simulink model "qss_saab93_optigear"  (Simulink 8.8)
settings: Solver=VariableStepDiscrete  StartTime=0.0  StopTime=1220  RelTol=1e-3  EnableMultiTasking=on
undefined symbols (not defined in the file or in its folder): g, h, rho
libraries: qss_tb_library x3
settings Model: Creator=grauers  LastModifiedBy=grauers
settings OptimizationCC: InitFltsAndDblsToZero=on
settings DebuggingCC: SaveWithParameterizedLinksMsg=none  SignalResolutionControl=TryResolveAllWithWarning  SolverPrmCheckMsg=warning  MultiTaskDSMMsg=warning  MultiTaskCondExecSysMsg=none  StateNameClashWarn=none  StrictBusMsg=None
settings GRTTargetCC: TargetFcnLib=ansi_tfl_tmw.mat  GeneratePreprocessorConditionals=Use local settings

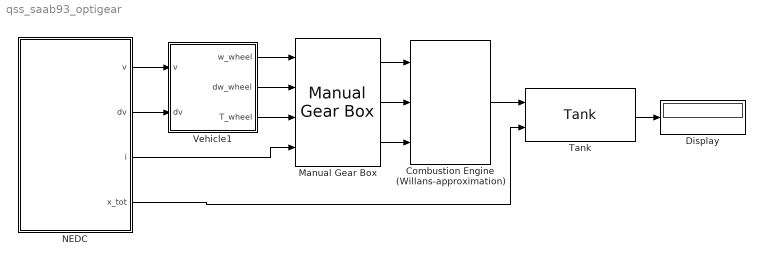
== system qss_saab93_optigear ==
  Combustion Engine (Willans-approximation) : qss_tb_library/Energy Converter/Combustion Engine (Willans-approximation)  Tag=combustion engine  engine_type=Otto  V_d=1.985  theta_CE=0.05  S=78  B=90  w_CE_idle=105  P_CE_idle=2600  P_aux=300  e=0.46  PI=1.44  p_me0g=1  ENABLE_FUEL_CUTOFF=on  T_CE_cutoff=5  P_CE_cutoff=0
  Display : Display
  Manual Gear Box : qss_tb_library/Gear System/Manual Gear Box  Tag=transmission  i_1=first_gear  i_2=second_gear  i_3=third_gear  i_4=fourth_gear  i_5=fifth_gear  i_diff=diff_gear  e_GT=0.98  P_GT0=300  w_wheel_min=1
  NEDC : Subsystem  Tag=cycle  mask(Driving Cycle){cyclename1=NEDC, stepsize=1, autostop=on}
      mask prompts: cyclename1 "Choose a cycle"; stepsize "Step size [s]"; autostop "Enable automatic simulation stop"
      mask help:
      | This block loads the cycle data such as time, speed, acceleration and gear number,  from the specified data file and makes it available on the output of the cycle block.
      |
      | Output:
      | ======
      | 	v	Speed [m/s]
      | 	dv	Acceleration [m/s^2]
      | 	i	Gear number [-]
      | 	x_tot	Total distance [m]
      |
      | Tip:
      | ===
      | Probably you don't need the gear number "i". If so you can terminate
      | it with a "Terminator" out of the "Simulink Library/Connections."
      |
      | Driving cycle:
      | ===
      | Select a driving cycle from the list below or specify your own (place your .mat file in the
      | directory Data/DrivingCycles/UserDefined)
      |
      | ECE_MAN
      | ECE_R15s
      | ECE_R15
      | EUDC
      | EUDC_MAN
      | City
      | City_MAN
      | NEDC
      | NEDC_MANl
      | GOT1
      | GOT2
      | GOT3
      | 10_15_MODE
      | 10_MODE
      | 10_MODE_3
      | 11_MODE
      | 11_MODE_4
      | 15_MODE
      | City_I
      | City_II
      | FTP_75
      | FTP_Highway
      |
      |
      | Step size:
      | ========
      | Default value is 1. Don't change it, unless you are familiar with the programs of the QSS TB.
      |
      | Enable automatic simulation stop:
      | ===========================
      | Stops the simulation automatically at the end of the cycle.
      | Be careful: If you have a component in your model that has to run after the cycle has finished, e.g. a battery to charge, remove the mark!
      mask init:
      | init_driving_cycle1;
      mask Display: plot(T_zplot, V_zplot);
  Tank : qss_tb_library/Energy Source/Tank  Tag=tank  fuel=Gasoline  flag_cold_start=on
  Vehicle1 : Subsystem  Tag=vehicle  mask(Vehicle){m_f=1295+80+100, mt2m_f=5, A_f=2, d_wheel=0.62, cw=0.3, mu=0.013}
      mask prompts: m_f "Total mass of the vehicle [kg]"; mt2m_f "Rotating mass [%]"; A_f "Vehicle cross section [m^2]"; d_wheel "Wheel diameter [m]"; cw "Drag coefficient [-]"; mu "Rolling friction coefficient [-]"
      mask help:
      | This block computes the power required from the vehicle.
      |
      | Input:
      | =====
      | 	v		Speed [m/s]
      | 	dv		Acceleration [m/s^2]
      |
      | Output:
      | ======
      | 	w_wheel	Speed of the wheel [rad/s]
      | 	dw_wheel	Acceleration of the wheel [rad/s^2]
      | 	T_wheel	Torque on the wheel [Nm]
      mask init:
      | init_vehicle;
  wires:
  NEDC/1(v) -> Vehicle1/1(v)
  Vehicle1/1(w_wheel) -> Manual Gear Box/1
  Vehicle1/2(dw_wheel) -> Manual Gear Box/2
  Vehicle1/3(T_wheel) -> Manual Gear Box/3
  NEDC/2(dv) -> Vehicle1/2(dv)
  Manual Gear Box/1 -> Combustion Engine (Willans-approximation)/1
  Manual Gear Box/2 -> Combustion Engine (Willans-approximation)/2
  Manual Gear Box/3 -> Combustion Engine (Willans-approximation)/3
  Combustion Engine (Willans-approximation)/1 -> Tank/1
  NEDC/3(i) -> Manual Gear Box/4
  NEDC/4(x_tot) -> Tank/2
  Tank/1 -> Display/1

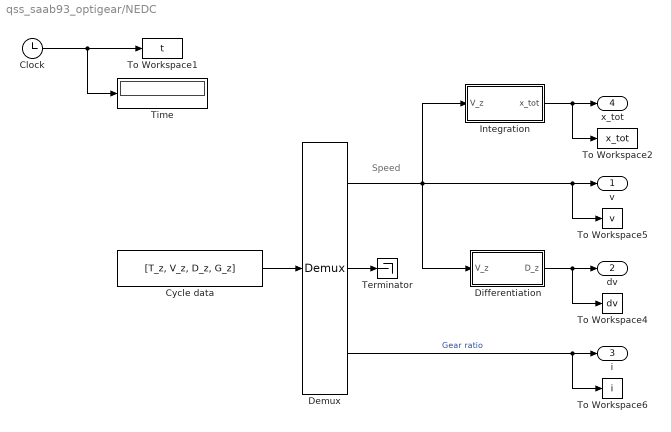
== system qss_saab93_optigear/NEDC ==
  note: Speed
  Clock : Clock
  Cycle data : FromWorkspace  VariableName=[T_z, V_z, D_z, G_z]  SampleTime=h
  Demux : Demux  Outputs=3
  Differentiation : Subsystem
  Integration : Subsystem
  Terminator : Terminator
  Time : Display
  To Workspace1 : ToWorkspace  VariableName=t  SampleTime=-1
  To Workspace2 : ToWorkspace  VariableName=x_tot  SampleTime=-1
  To Workspace4 : ToWorkspace  VariableName=dv  SampleTime=-1
  To Workspace5 : ToWorkspace  VariableName=v  SampleTime=-1
  To Workspace6 : ToWorkspace  VariableName=i  SampleTime=-1
  v : Outport  InitialOutput=0
  dv : Outport  Port=2  InitialOutput=0
  i : Outport  Port=3  InitialOutput=0
  x_tot : Outport  Port=4  InitialOutput=0
  wires:
  Clock/1 -> To Workspace1/1, Time/1
  Demux/3 -> To Workspace6/1, i/1  "Gear ratio"
  Integration/1(x_tot) -> To Workspace2/1, x_tot/1
  Demux/1 -> Differentiation/1(V_z), To Workspace5/1, v/1, Integration/1(V_z)
  Demux/2 -> Terminator/1
  Differentiation/1(D_z) -> dv/1, To Workspace4/1
  Cycle data/1 -> Demux/1

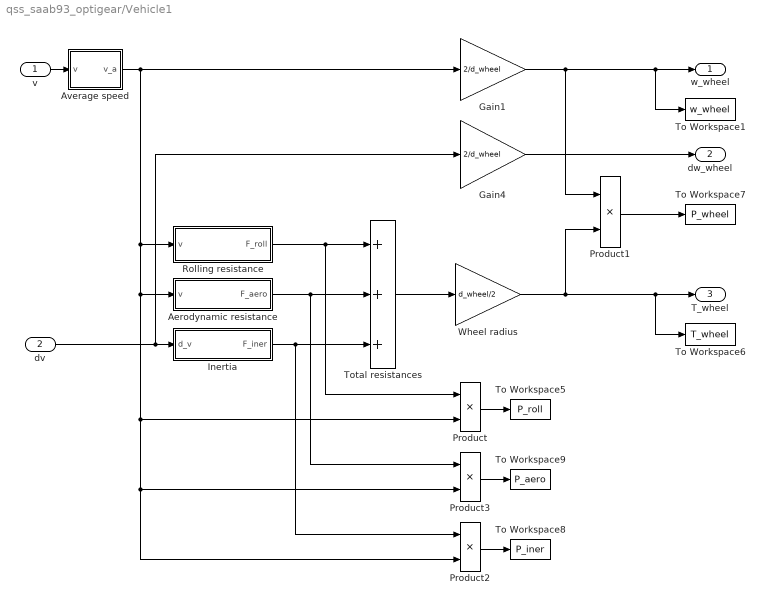
== system qss_saab93_optigear/Vehicle1 ==
  v : Inport
  dv : Inport  Port=2
  Aerodynamic resistance : Subsystem
  Average speed : Subsystem
  Gain1 : Gain  Gain=2/d_wheel  SaturateOnIntegerOverflow=on  OutDataTypeStr=Inherit: Same as input  ParamDataTypeStr=Inherit: Same as input
  Gain4 : Gain  Gain=2/d_wheel  SaturateOnIntegerOverflow=on  OutDataTypeStr=Inherit: Same as input  ParamDataTypeStr=Inherit: Same as input
  Inertia : Subsystem
  Product{,1..3} (4 alike) : Product  SaturateOnIntegerOverflow=on  RndMeth=Zero  InputSameDT=on  OutDataTypeStr=Inherit: Same as first input
  Rolling resistance : Subsystem
  To Workspace1 : ToWorkspace  VariableName=w_wheel  SampleTime=-1
  To Workspace5 : ToWorkspace  VariableName=P_roll  SampleTime=-1
  To Workspace6 : ToWorkspace  VariableName=T_wheel  SampleTime=-1
  To Workspace7 : ToWorkspace  VariableName=P_wheel  SampleTime=-1
  To Workspace8 : ToWorkspace  VariableName=P_iner  SampleTime=-1
  To Workspace9 : ToWorkspace  VariableName=P_aero  SampleTime=-1
  Total resistances : Sum  Inputs=+++  SaturateOnIntegerOverflow=on  InputSameDT=on  OutDataTypeStr=Inherit: Same as first input
  Wheel radius : Gain  Gain=d_wheel/2  SaturateOnIntegerOverflow=on  OutDataTypeStr=Inherit: Same as input  ParamDataTypeStr=Inherit: Same as input
  w_wheel : Outport  InitialOutput=0
  dw_wheel : Outport  Port=2  InitialOutput=0
  T_wheel : Outport  Port=3  InitialOutput=0
  wires:
  Gain4/1 -> dw_wheel/1
  Gain1/1 -> Product1/1, w_wheel/1, To Workspace1/1
  Rolling resistance/1(F_roll) -> Total resistances/1, Product/1
  Aerodynamic resistance/1(F_aero) -> Product3/1, Total resistances/2
  Inertia/1(F_iner) -> Total resistances/3, Product2/1
  Total resistances/1 -> Wheel radius/1
  Wheel radius/1 -> Product1/2, T_wheel/1, To Workspace6/1
  Average speed/1(v_a) -> Gain1/1, Aerodynamic resistance/1(v), Product/2, Product3/2, Product2/2, Rolling resistance/1(v)
  dv/1 -> Inertia/1(d_v), Gain4/1
  v/1 -> Average speed/1(v)
  Product2/1 -> To Workspace8/1
  Product3/1 -> To Workspace9/1
  Product1/1 -> To Workspace7/1
  Product/1 -> To Workspace5/1

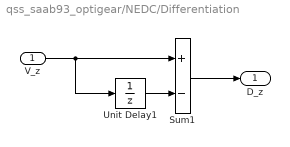
== system qss_saab93_optigear/NEDC/Differentiation ==
  V_z : Inport
  Sum1 : Sum  Inputs=+-  SaturateOnIntegerOverflow=on  InputSameDT=on  OutDataTypeStr=Inherit: Same as first input
  Unit Delay1 : UnitDelay  SampleTime=h
  D_z : Outport  InitialOutput=0
  wires:
  Sum1/1 -> D_z/1
  V_z/1 -> Unit Delay1/1, Sum1/1
  Unit Delay1/1 -> Sum1/2

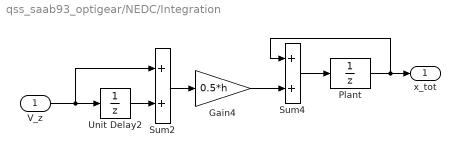
== system qss_saab93_optigear/NEDC/Integration ==
  V_z : Inport
  Gain4 : Gain  Gain=0.5*h  SaturateOnIntegerOverflow=on  OutDataTypeStr=Inherit: Same as input  ParamDataTypeStr=Inherit: Same as input
  Plant : UnitDelay  InitialCondition=1  SampleTime=h
  Sum2 : Sum  SaturateOnIntegerOverflow=on  InputSameDT=on  OutDataTypeStr=Inherit: Same as first input
  Sum4 : Sum  SaturateOnIntegerOverflow=on  InputSameDT=on  OutDataTypeStr=Inherit: Same as first input
  Unit Delay2 : UnitDelay  SampleTime=h
  x_tot : Outport  InitialOutput=0
  wires:
  Plant/1 -> x_tot/1, Sum4/1
  Sum4/1 -> Plant/1
  Gain4/1 -> Sum4/2
  V_z/1 -> Unit Delay2/1, Sum2/1
  Unit Delay2/1 -> Sum2/2
  Sum2/1 -> Gain4/1

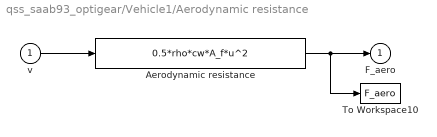
== system qss_saab93_optigear/Vehicle1/Aerodynamic resistance ==
  v : Inport
  Aerodynamic resistance : Fcn  Expr=0.5*rho*cw*A_f*u^2
  To Workspace10 : ToWorkspace  VariableName=F_aero  SampleTime=-1
  F_aero : Outport  InitialOutput=0
  wires:
  v/1 -> Aerodynamic resistance/1
  Aerodynamic resistance/1 -> F_aero/1, To Workspace10/1

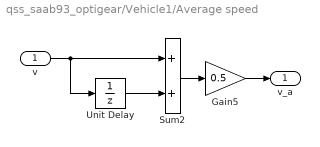
== system qss_saab93_optigear/Vehicle1/Average speed ==
  v : Inport
  Gain5 : Gain  Gain=0.5  SaturateOnIntegerOverflow=on  OutDataTypeStr=Inherit: Same as input  ParamDataTypeStr=Inherit: Same as input
  Sum2 : Sum  SaturateOnIntegerOverflow=on  InputSameDT=on  OutDataTypeStr=Inherit: Same as first input
  Unit Delay : UnitDelay  SampleTime=h
  v_a : Outport  InitialOutput=0
  wires:
  Unit Delay/1 -> Sum2/2
  Sum2/1 -> Gain5/1
  Gain5/1 -> v_a/1
  v/1 -> Sum2/1, Unit Delay/1

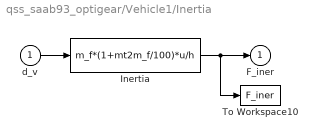
== system qss_saab93_optigear/Vehicle1/Inertia ==
  d_v : Inport
  Inertia : Fcn  Expr=m_f*(1+mt2m_f/100)*u/h
  To Workspace10 : ToWorkspace  VariableName=F_iner  SampleTime=-1
  F_iner : Outport  InitialOutput=0
  wires:
  Inertia/1 -> F_iner/1, To Workspace10/1
  d_v/1 -> Inertia/1

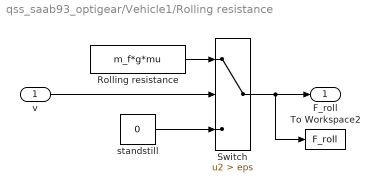
== system qss_saab93_optigear/Vehicle1/Rolling resistance ==
  v : Inport
  Rolling resistance : Constant  Value=m_f*g*mu
  Switch : Switch  Criteria=u2 > Threshold  Threshold=eps
  To Workspace2 : ToWorkspace  VariableName=F_roll  SampleTime=-1
  standstill : Constant  Value=0
  F_roll : Outport
  wires:
  Switch/1 -> To Workspace2/1, F_roll/1
  v/1 -> Switch/2
  standstill/1 -> Switch/3
  Rolling resistance/1 -> Switch/1
